simulink model "Actuators_Model"  (R2015a)
settings: Solver=ode45  StartTime=0.0  StopTime=10  RelTol=1e-3
values from neighbouring files (symbols this model uses):
  b = 0.55/2    (= 0.275)    [TiltCopter_Parameters.m]
  B0 = 1.399e04    (= 13990)    [TiltCopter_Parameters.m]
  B1 = 1150    [TiltCopter_Parameters.m]
  B2 = 37.46    [TiltCopter_Parameters.m]
  B3 = 1    [TiltCopter_Parameters.m]
  degtorad = pi/180    (= 0.0174532925199)    [TiltCopter_Parameters.m]
  Kq = Cq*ro*A*R^3    (= 2.88925724261e-07)    [TiltCopter_Parameters.m]
  Kt = Ct*ro*A*R^2    (= 2.46191978476e-05)    [TiltCopter_Parameters.m]
  m_servo = p(1)    [TiltCopter_Parameters.m]
  q_servo = p(2)    [TiltCopter_Parameters.m]
  ServoMotor_Gain = 1.409e04    (= 14090)    [TiltCopter_Parameters.m]
  tau = 0.055257    [TiltCopter_Parameters.m]
  x1 = [m q]    [TiltCopter_Parameters.m]
settings Model: Creator=Claudio  LastModifiedBy=Claudio

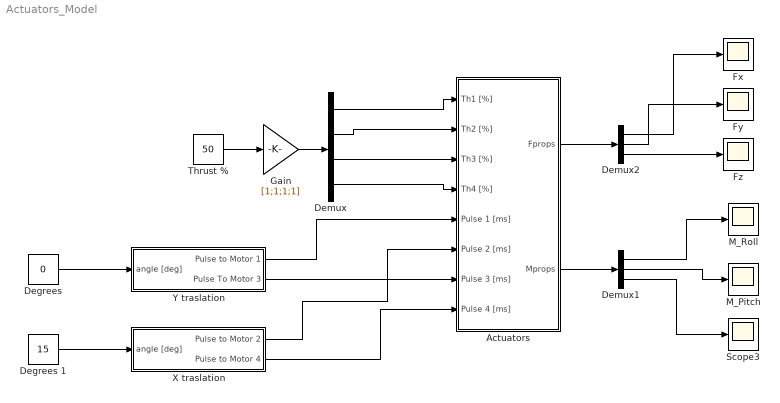
== system Actuators_Model ==
  Actuators : Subsystem
  "Degrees " : Constant  Value=0
  Degrees 1 : Constant  Value=15
  Demux : Demux
  Demux1 : Demux  Outputs=3
  Demux2 : Demux  Outputs=3
  Fx : Scope
      settings: SaveName=ScopeData2
  Fy : Scope
      settings: YMin=-6  YMax=8
  Fz : Scope
      settings: YMin=-25  YMax=0
  Gain : Gain  Gain=[1;1;1;1]
  M_Pitch : Scope
      settings: YMin=-6  YMax=8  SaveName=ScopeData4
  M_Roll : Scope
      settings: SaveName=ScopeData5
  Scope3 : Scope
      settings: YMin=-25  YMax=0  SaveName=ScopeData3
  Thrust % : Constant  Value=50
  X traslation : Subsystem
  Y traslation : Subsystem
  wires:
  Thrust %/1 -> Gain/1
  Gain/1 -> Demux/1
  Demux/1 -> Actuators/1(Th1 [%])
  Demux/2 -> Actuators/2(Th2 [%])
  Demux/3 -> Actuators/3(Th3 [%])
  Demux/4 -> Actuators/4(Th4 [%])
  Actuators/1(Fprops) -> Demux2/1
  Demux2/3 -> Fz/1
  Demux2/1 -> Fx/1
  Demux2/2 -> Fy/1
  "Degrees "/1 -> Y traslation/1(angle [deg])
  Y traslation/1(Pulse to Motor 1) -> Actuators/5(Pulse 1 [ms])
  Y traslation/2(Pulse To Motor 3) -> Actuators/7(Pulse 3 [ms])
  Degrees 1/1 -> X traslation/1(angle [deg])
  X traslation/1(Pulse to Motor 2) -> Actuators/6(Pulse 2 [ms])
  X traslation/2(Pulse to Motor 4) -> Actuators/8(Pulse 4 [ms])
  Actuators/2(Mprops) -> Demux1/1
  Demux1/3 -> Scope3/1
  Demux1/1 -> M_Roll/1
  Demux1/2 -> M_Pitch/1

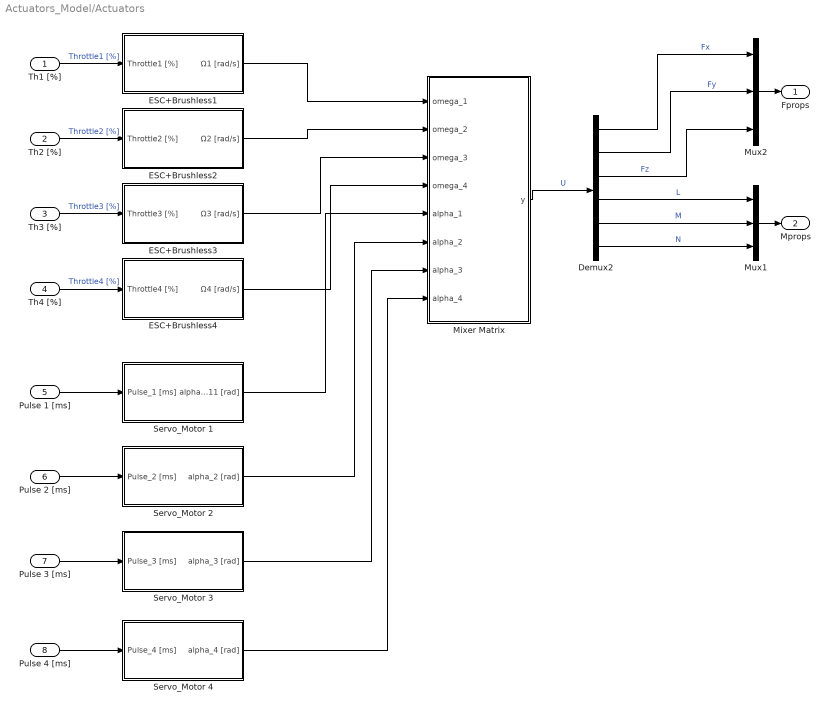
== system Actuators_Model/Actuators ==
  Th1 [%] : Inport
  Th2 [%] : Inport  Port=2
  Th3 [%] : Inport  Port=3
  Th4 [%] : Inport  Port=4
  Pulse 1 [ms] : Inport  Port=5
  Pulse 2 [ms] : Inport  Port=6
  Pulse 3 [ms] : Inport  Port=7
  Pulse 4 [ms] : Inport  Port=8
  Demux2 : Demux  Outputs=6
  ESC+Brushless1 : Subsystem
  ESC+Brushless2 : Subsystem
  ESC+Brushless3 : Subsystem
  ESC+Brushless4 : Subsystem
  Mixer Matrix : MATLAB Function  TreatAsAtomicUnit=on
  Mux1 : Mux  Inputs=3
  Mux2 : Mux  Inputs=3
  Servo_Motor 1 : Subsystem
  Servo_Motor 2 : Subsystem
  Servo_Motor 3 : Subsystem
  Servo_Motor 4 : Subsystem
  Fprops : Outport
  Mprops : Outport  Port=2
  wires:
  Mixer Matrix/1(y) -> Demux2/1  "U"
  Th1 [%]/1 -> ESC+Brushless1/1(Throttle1 [%])  "Throttle1 [%]"
  Th2 [%]/1 -> ESC+Brushless2/1(Throttle2 [%])  "Throttle2 [%]"
  Th4 [%]/1 -> ESC+Brushless4/1(Throttle4 [%])  "Throttle4 [%]"
  Th3 [%]/1 -> ESC+Brushless3/1(Throttle3 [%])  "Throttle3 [%]"
  Mux1/1 -> Mprops/1
  Mux2/1 -> Fprops/1
  Pulse 1 [ms]/1 -> Servo_Motor 1/1(Pulse_1 [ms])
  Pulse 2 [ms]/1 -> Servo_Motor 2/1(Pulse_2 [ms])
  Pulse 3 [ms]/1 -> Servo_Motor 3/1(Pulse_3 [ms])
  Pulse 4 [ms]/1 -> Servo_Motor 4/1(Pulse_4 [ms])
  ESC+Brushless1/1(Ω1 [rad/s]) -> Mixer Matrix/1(omega_1)
  ESC+Brushless2/1(Ω2 [rad/s]) -> Mixer Matrix/2(omega_2)
  ESC+Brushless3/1(Ω3 [rad/s]) -> Mixer Matrix/3(omega_3)
  ESC+Brushless4/1(Ω4 [rad/s]) -> Mixer Matrix/4(omega_4)
  Servo_Motor 2/1(alpha_2 [rad]) -> Mixer Matrix/6(alpha_2)
  Servo_Motor 3/1(alpha_3 [rad]) -> Mixer Matrix/7(alpha_3)
  Servo_Motor 4/1(alpha_4 [rad]) -> Mixer Matrix/8(alpha_4)
  Demux2/1 -> Mux2/1  "Fx"
  Demux2/2 -> Mux2/2  "Fy"
  Demux2/3 -> Mux2/3  "Fz"
  Demux2/4 -> Mux1/1  "L"
  Demux2/5 -> Mux1/2  "M"
  Demux2/6 -> Mux1/3  "N"
  Servo_Motor 1/1(alpha_11 [rad]) -> Mixer Matrix/5(alpha_1)

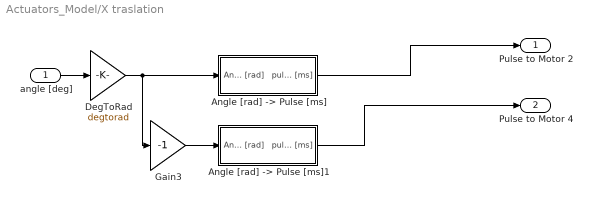
== system Actuators_Model/X traslation ==
  angle [deg] : Inport
  "Angle [rad] -> Pulse [ms]" : Subsystem
  "Angle [rad] -> Pulse [ms]1" : Subsystem
  DegToRad : Gain  Gain=degtorad
  Gain3 : Gain  Gain=-1
  Pulse to Motor 2 : Outport
  Pulse to Motor 4 : Outport  Port=2
  wires:
  "Angle [rad] -> Pulse [ms]1"/1(pulse [ms]) -> Pulse to Motor 4/1
  Gain3/1 -> "Angle [rad] -> Pulse [ms]1"/1(Angle [rad])
  angle [deg]/1 -> DegToRad/1
  DegToRad/1 -> "Angle [rad] -> Pulse [ms]"/1(Angle [rad]), Gain3/1
  "Angle [rad] -> Pulse [ms]"/1(pulse [ms]) -> Pulse to Motor 2/1

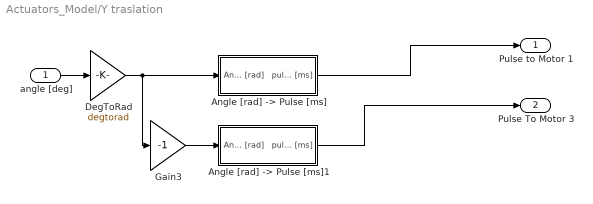
== system Actuators_Model/Y traslation ==
  angle [deg] : Inport
  "Angle [rad] -> Pulse [ms]" : Subsystem
  "Angle [rad] -> Pulse [ms]1" : Subsystem
  DegToRad : Gain  Gain=degtorad
  Gain3 : Gain  Gain=-1
  Pulse to Motor 1 : Outport
  Pulse To Motor 3 : Outport  Port=2
  wires:
  "Angle [rad] -> Pulse [ms]1"/1(pulse [ms]) -> Pulse To Motor 3/1
  Gain3/1 -> "Angle [rad] -> Pulse [ms]1"/1(Angle [rad])
  angle [deg]/1 -> DegToRad/1
  DegToRad/1 -> Gain3/1, "Angle [rad] -> Pulse [ms]"/1(Angle [rad])
  "Angle [rad] -> Pulse [ms]"/1(pulse [ms]) -> Pulse to Motor 1/1

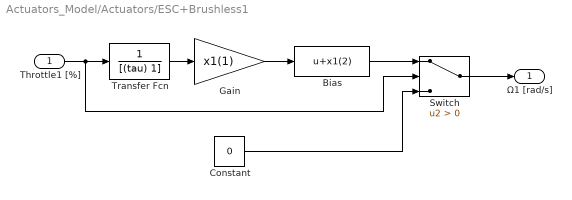
== system Actuators_Model/Actuators/ESC+Brushless1 ==
  Throttle1 [%] : Inport
  Bias : Bias  Bias=x1(2)
  Constant : Constant  Value=0
  Gain : Gain  Gain=x1(1)
  Switch : Switch  Criteria=u2 > Threshold
  Transfer Fcn : TransferFcn  Denominator=[(tau) 1]
  Ω1 [rad/s] : Outport
  wires:
  Gain/1 -> Bias/1
  Bias/1 -> Switch/1
  Constant/1 -> Switch/3
  Switch/1 -> Ω1 [rad/s]/1
  Throttle1 [%]/1 -> Transfer Fcn/1, Switch/2
  Transfer Fcn/1 -> Gain/1

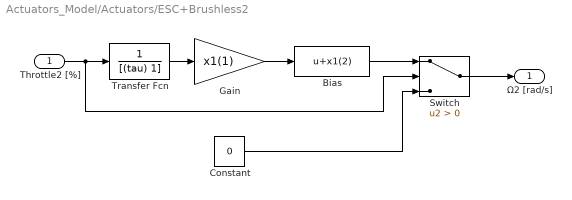
== system Actuators_Model/Actuators/ESC+Brushless2 ==
  Throttle2 [%] : Inport
  Bias : Bias  Bias=x1(2)
  Constant : Constant  Value=0
  Gain : Gain  Gain=x1(1)
  Switch : Switch  Criteria=u2 > Threshold
  Transfer Fcn : TransferFcn  Denominator=[(tau) 1]
  Ω2 [rad/s] : Outport
  wires:
  Switch/1 -> Ω2 [rad/s]/1
  Constant/1 -> Switch/3
  Bias/1 -> Switch/1
  Gain/1 -> Bias/1
  Throttle2 [%]/1 -> Transfer Fcn/1, Switch/2
  Transfer Fcn/1 -> Gain/1

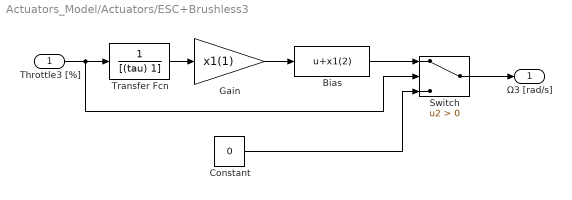
== system Actuators_Model/Actuators/ESC+Brushless3 ==
  Throttle3 [%] : Inport
  Bias : Bias  Bias=x1(2)
  Constant : Constant  Value=0
  Gain : Gain  Gain=x1(1)
  Switch : Switch  Criteria=u2 > Threshold
  Transfer Fcn : TransferFcn  Denominator=[(tau) 1]
  Ω3 [rad/s] : Outport
  wires:
  Gain/1 -> Bias/1
  Bias/1 -> Switch/1
  Constant/1 -> Switch/3
  Switch/1 -> Ω3 [rad/s]/1
  Throttle3 [%]/1 -> Transfer Fcn/1, Switch/2
  Transfer Fcn/1 -> Gain/1

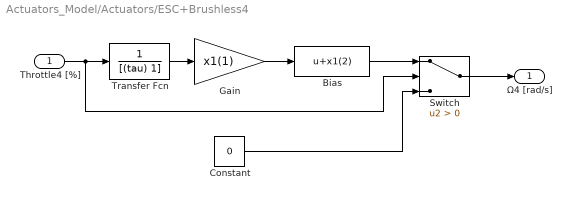
== system Actuators_Model/Actuators/ESC+Brushless4 ==
  Throttle4 [%] : Inport
  Bias : Bias  Bias=x1(2)
  Constant : Constant  Value=0
  Gain : Gain  Gain=x1(1)
  Switch : Switch  Criteria=u2 > Threshold
  Transfer Fcn : TransferFcn  Denominator=[(tau) 1]
  Ω4 [rad/s] : Outport
  wires:
  Switch/1 -> Ω4 [rad/s]/1
  Constant/1 -> Switch/3
  Bias/1 -> Switch/1
  Gain/1 -> Bias/1
  Throttle4 [%]/1 -> Transfer Fcn/1, Switch/2
  Transfer Fcn/1 -> Gain/1

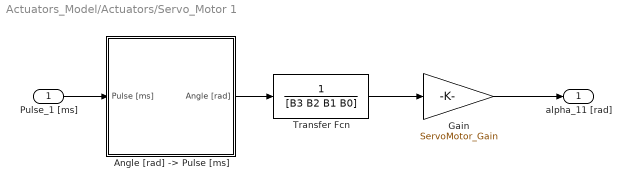
== system Actuators_Model/Actuators/Servo_Motor 1 ==
  Pulse_1 [ms] : Inport
  "Angle [rad] -> Pulse [ms]" : Subsystem
  Gain : Gain  Gain=ServoMotor_Gain
  Transfer Fcn : TransferFcn  Denominator=[B3 B2 B1 B0]
  alpha_11 [rad] : Outport
  wires:
  Gain/1 -> alpha_11 [rad]/1
  Transfer Fcn/1 -> Gain/1
  "Angle [rad] -> Pulse [ms]"/1(Angle [rad]) -> Transfer Fcn/1
  Pulse_1 [ms]/1 -> "Angle [rad] -> Pulse [ms]"/1(Pulse [ms])

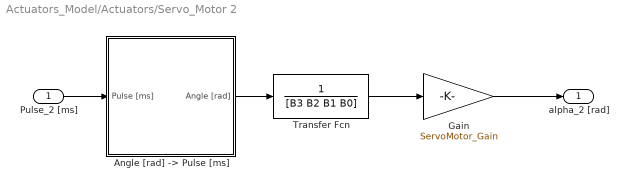
== system Actuators_Model/Actuators/Servo_Motor 2 ==
  Pulse_2 [ms] : Inport
  "Angle [rad] -> Pulse [ms]" : Subsystem
  Gain : Gain  Gain=ServoMotor_Gain
  Transfer Fcn : TransferFcn  Denominator=[B3 B2 B1 B0]
  alpha_2 [rad] : Outport
  wires:
  Gain/1 -> alpha_2 [rad]/1
  Transfer Fcn/1 -> Gain/1
  "Angle [rad] -> Pulse [ms]"/1(Angle [rad]) -> Transfer Fcn/1
  Pulse_2 [ms]/1 -> "Angle [rad] -> Pulse [ms]"/1(Pulse [ms])

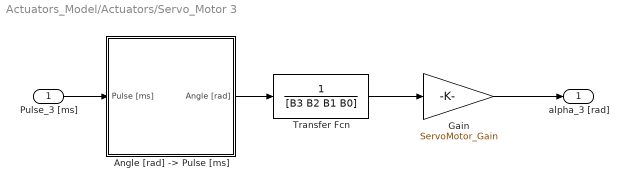
== system Actuators_Model/Actuators/Servo_Motor 3 ==
  Pulse_3 [ms] : Inport
  "Angle [rad] -> Pulse [ms]" : Subsystem
  Gain : Gain  Gain=ServoMotor_Gain
  Transfer Fcn : TransferFcn  Denominator=[B3 B2 B1 B0]
  alpha_3 [rad] : Outport
  wires:
  Gain/1 -> alpha_3 [rad]/1
  Transfer Fcn/1 -> Gain/1
  "Angle [rad] -> Pulse [ms]"/1(Angle [rad]) -> Transfer Fcn/1
  Pulse_3 [ms]/1 -> "Angle [rad] -> Pulse [ms]"/1(Pulse [ms])

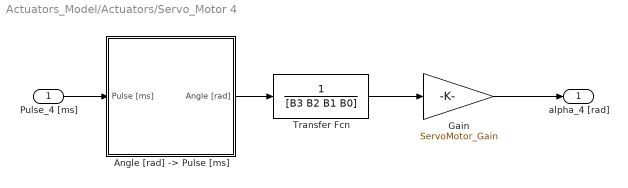
== system Actuators_Model/Actuators/Servo_Motor 4 ==
  Pulse_4 [ms] : Inport
  "Angle [rad] -> Pulse [ms]" : Subsystem
  Gain : Gain  Gain=ServoMotor_Gain
  Transfer Fcn : TransferFcn  Denominator=[B3 B2 B1 B0]
  alpha_4 [rad] : Outport
  wires:
  Gain/1 -> alpha_4 [rad]/1
  Transfer Fcn/1 -> Gain/1
  "Angle [rad] -> Pulse [ms]"/1(Angle [rad]) -> Transfer Fcn/1
  Pulse_4 [ms]/1 -> "Angle [rad] -> Pulse [ms]"/1(Pulse [ms])

== system Actuators_Model/X traslation/Angle [rad] -> Pulse [ms] ==
  Angle [rad] : Inport
  Add : Sum
  Constant : Constant  Value=q_servo
  Linear fitting gain : Gain  Gain=m_servo
  pulse [ms] : Outport
  wires:
  Angle [rad]/1 -> Linear fitting gain/1
  Constant/1 -> Add/2
  Linear fitting gain/1 -> Add/1
  Add/1 -> pulse [ms]/1

== system Actuators_Model/X traslation/Angle [rad] -> Pulse [ms]1 ==
  Angle [rad] : Inport
  Add : Sum
  Constant : Constant  Value=q_servo
  Linear fitting gain : Gain  Gain=m_servo
  pulse [ms] : Outport
  wires:
  Angle [rad]/1 -> Linear fitting gain/1
  Constant/1 -> Add/2
  Linear fitting gain/1 -> Add/1
  Add/1 -> pulse [ms]/1

== system Actuators_Model/Y traslation/Angle [rad] -> Pulse [ms] ==
  Angle [rad] : Inport
  Add : Sum
  Constant : Constant  Value=q_servo
  Linear fitting gain : Gain  Gain=m_servo
  pulse [ms] : Outport
  wires:
  Angle [rad]/1 -> Linear fitting gain/1
  Constant/1 -> Add/2
  Linear fitting gain/1 -> Add/1
  Add/1 -> pulse [ms]/1

== system Actuators_Model/Y traslation/Angle [rad] -> Pulse [ms]1 ==
  Angle [rad] : Inport
  Add : Sum
  Constant : Constant  Value=q_servo
  Linear fitting gain : Gain  Gain=m_servo
  pulse [ms] : Outport
  wires:
  Add/1 -> pulse [ms]/1
  Linear fitting gain/1 -> Add/1
  Constant/1 -> Add/2
  Angle [rad]/1 -> Linear fitting gain/1

== system Actuators_Model/Actuators/Servo_Motor 1/Angle [rad] -> Pulse [ms] ==
  Pulse [ms] : Inport
  Add : Sum  Inputs=+-
  Constant : Constant  Value=q_servo
  Linear fitting gain : Gain  Gain=1/m_servo
  Angle [rad] : Outport
  wires:
  Constant/1 -> Add/2
  Add/1 -> Linear fitting gain/1
  Pulse [ms]/1 -> Add/1
  Linear fitting gain/1 -> Angle [rad]/1

== system Actuators_Model/Actuators/Servo_Motor 2/Angle [rad] -> Pulse [ms] ==
  Pulse [ms] : Inport
  Add : Sum  Inputs=+-
  Constant : Constant  Value=q_servo
  Linear fitting gain : Gain  Gain=1/m_servo
  Angle [rad] : Outport
  wires:
  Constant/1 -> Add/2
  Add/1 -> Linear fitting gain/1
  Pulse [ms]/1 -> Add/1
  Linear fitting gain/1 -> Angle [rad]/1

== system Actuators_Model/Actuators/Servo_Motor 3/Angle [rad] -> Pulse [ms] ==
  Pulse [ms] : Inport
  Add : Sum  Inputs=+-
  Constant : Constant  Value=q_servo
  Linear fitting gain : Gain  Gain=1/m_servo
  Angle [rad] : Outport
  wires:
  Constant/1 -> Add/2
  Add/1 -> Linear fitting gain/1
  Pulse [ms]/1 -> Add/1
  Linear fitting gain/1 -> Angle [rad]/1

== system Actuators_Model/Actuators/Servo_Motor 4/Angle [rad] -> Pulse [ms] ==
  Pulse [ms] : Inport
  Add : Sum  Inputs=+-
  Constant : Constant  Value=q_servo
  Linear fitting gain : Gain  Gain=1/m_servo
  Angle [rad] : Outport
  wires:
  Constant/1 -> Add/2
  Add/1 -> Linear fitting gain/1
  Pulse [ms]/1 -> Add/1
  Linear fitting gain/1 -> Angle [rad]/1

== matlab function Actuators_Model/Actuators/Mixer Matrix ==
  data: omega_1 input; y output; omega_2 input; omega_3 input; omega_4 input; alpha_1 input; alpha_2 input; alpha_3 input; alpha_4 input; Kt parameter; Kq parameter; b parameter
function y = fcn(omega_1,omega_2,omega_3,omega_4,alpha_1,alpha_2,alpha_3,alpha_4,Kt,Kq,b)
%#codegen


% F_ext comumns are [Fx;Fy;Fz]
F_ext =[ Kt*sin(alpha_2)*omega_2^2 - Kt*sin(alpha_4)*omega_4^2;
         - Kt*sin(alpha_1)*omega_1^2 + Kt*sin(alpha_3)*omega_3^2;
         - Kt*cos(alpha_1)*omega_1^2 - Kt*cos(alpha_2)*omega_2^2 - Kt*cos(alpha_3)*omega_3^2 - Kt*cos(alpha_4)*omega_4^2 
        ];

% M_ext colums are [M_roll;M_Pitch;M_yaw]    
M_ext =[ Kq*omega_2^2*sin(alpha_2) - Kq*omega_4^2*sin(alpha_4) - Kt*b*omega_2^2*cos(alpha_2) + Kt*b*omega_4^2*cos(alpha_4);
         Kq*omega_1^2*sin(alpha_1) - Kq*omega_3^2*sin(alpha_3) + Kt*b*omega_1^2*cos(alpha_1) - Kt*b*omega_3^2*cos(alpha_3);
         Kq*omega_1^2*cos(alpha_1) - Kq*omega_2^2*cos(alpha_2) + Kq*omega_3^2*cos(alpha_3) - Kq*omega_4^2*cos(alpha_4) - Kt*b*omega_1^2*sin(alpha_1) - Kt*b*omega_2^2*sin(alpha_2) - Kt*b*omega_3^2*sin(alpha_3) - Kt*b*omega_4^2*sin(alpha_4);
       ];
 

y = [F_ext;M_ext];
